simulink model "Damper"  (R2021b)
settings: Solver=ode1  StartTime=0.0  StopTime=inf  FixedStep=0.001  RelTol=1e-3
settings Model: Creator=jalfonso  LastModifiedBy=au602135
settings SolverCC: AlgebraicLoopSolver=TrustRegion
settings DataIOCC: ReturnWorkspaceOutputs=off
settings DebuggingCC: SFMachineParentedDataDiag=warning  ArithmeticOperatorsInVariantConditions=warning
settings SFSimCC: SimUseLocalCustomCode=off  CustomCodeUndefinedFunction=UseInterfaceOnly
settings RTWCC: RTWUseLocalCustomCode=off
settings CodeAppCC: StateflowObjectComments=on

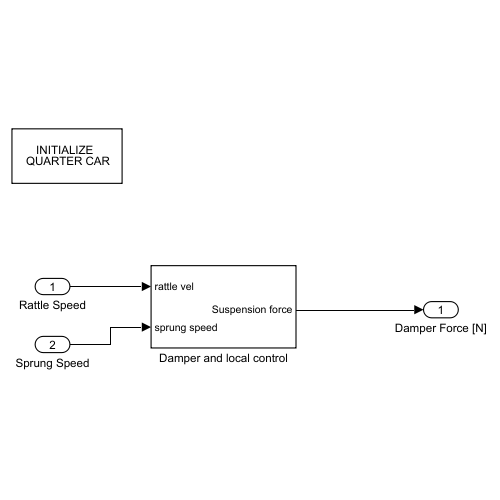
[thumbnail: Simulink's stored preview of the top-level diagram]
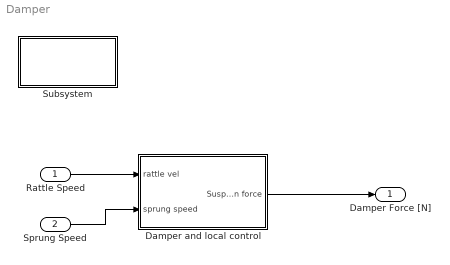
== system Damper ==
  Rattle Speed : Inport
  Sprung Speed : Inport  Port=2
  Damper and local control : Subsystem
  Subsystem : Subsystem
      settings: OpenFcn=|
      | k_tire = 225400;  %200000 in literature
      | c_tire = 100;        % Estimated. In literatures 6N
      | k_susp =  25000;  % 15000 in literature
      | c_susp = 400;       %1429 Ns/m in literature
      | g = 0 % 9.8; Removed to avoid initialization problems
      | m_unsprung = 66;
      | m_sprung = 449.25;
      | X_sprung0  = .5;
      | X_unsprung0  = .1;
      | delayTimeCarToDamper =  0.002;
      | %InitQuarterCarCompensatorScript;
      | %Amplitude =.01;
      mask Display: disp('INITIALIZE \n QUARTER CAR')
  Damper Force [N] : Outport
  wires:
  Damper and local control/1(Suspension force) -> Damper Force [N]/1
  Rattle Speed/1 -> Damper and local control/1(rattle vel)
  Sprung Speed/1 -> Damper and local control/2(sprung speed)

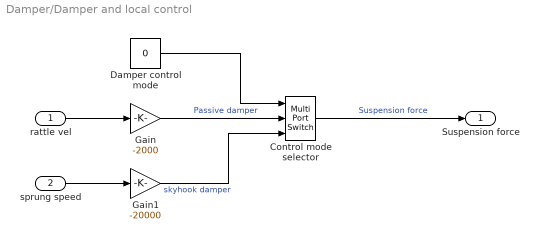
== system Damper/Damper and local control ==
  rattle vel : Inport
  sprung speed : Inport  Port=2
  Control mode selector : MultiPortSwitch  DataPortOrder=Zero-based contiguous  Inputs=2  zeroidx=on
  Damper control mode : Constant  Value=0
  Gain : Gain  Gain=-2000
  Gain1 : Gain  Gain=-20000
  Suspension force : Outport
  wires:
  Damper control mode/1 -> Control mode selector/1
  Gain1/1 -> Control mode selector/3  "skyhook damper"
  Gain/1 -> Control mode selector/2  "Passive damper"
  sprung speed/1 -> Gain1/1
  rattle vel/1 -> Gain/1
  Control mode selector/1 -> Suspension force/1  "Suspension force"

== system Damper/Subsystem ==
